simulink model "buckexp9"  (R2024b)
settings: Solver=ode4  StartTime=0.0  StopTime=0.05  FixedStep=1e-8  MaxStep=1e-4  RelTol=1e-3
libraries: spsVoltageMeasurementLib x4, spsSeriesRLCBranchLib x3, spsDiodeLib x1, spsCurrentMeasurementLib x1, spsMosfetLib x1, simulink x1, spsDCVoltageSourceLib x1, sps_lib x1
settings Model: Creator=ece  LastModifiedBy=User
settings SolverCC: AlgebraicLoopSolver=TrustRegion
settings DataIOCC: ReturnWorkspaceOutputs=off
settings DebuggingCC: UnconnectedInputMsg=warning  UnconnectedOutputMsg=warning  UnconnectedLineMsg=warning  ArithmeticOperatorsInVariantConditions=warning
settings ModelReferenceCC: EnableRefExpFcnMdlSchedulingChecks=on
settings SFSimCC: SimUseLocalCustomCode=off  CustomCodeUndefinedFunction=UseInterfaceOnly
settings RTWCC: RTWUseLocalCustomCode=off  GPUComputeCapability=3.5
settings CodeAppCC: StateflowObjectComments=on
settings SimscapeCC: SimscapeNormalizeSystem=off

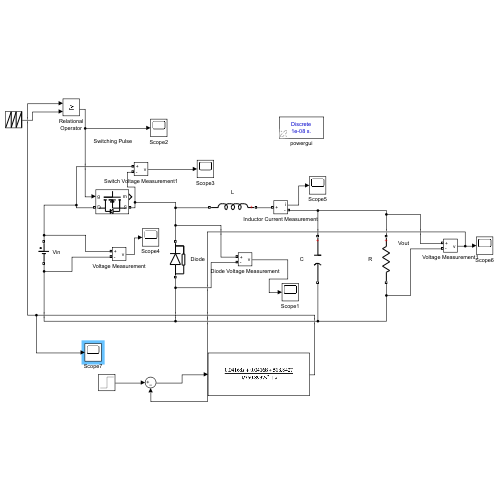
[thumbnail: Simulink's stored preview of the top-level diagram]
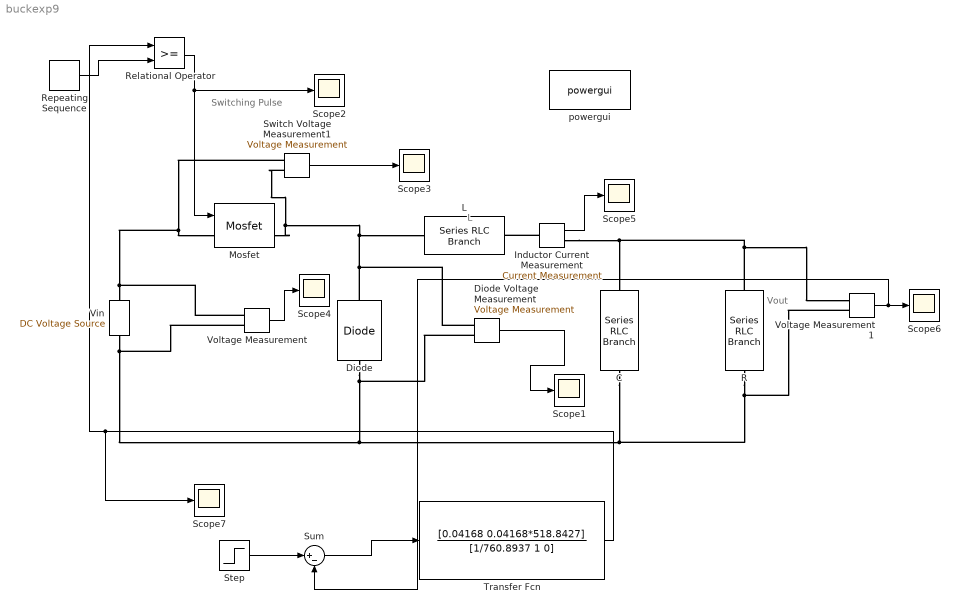
== system buckexp9 ==
  note: Vout
  note: Switching Pulse
  note: L
  "   C" : spsSeriesRLCBranchLib/Series RLC Branch  LConnTagsString=__new0  RConnTagsString=__new0  BranchType=C  Resistance=1  Inductance=1e-3  SetiL0=off  InitialCurrent=0  Capacitance=100e-6  Setx0=off  InitialVoltage=0  Measurements=None
  Diode : spsDiodeLib/Diode  Ron=0.001  Lon=0  Vf=0.8  IC=0  UseSnubber=0  Rs=5e5  Cs=250e-9  Measurements=off
  Diode Voltage Measurement : spsVoltageMeasurementLib/Voltage Measurement  PhasorSimulation=off  OutputType=Complex  PSBequivalent=0
  Inductor Current Measurement : spsCurrentMeasurementLib/Current Measurement  PhasorSimulation=off  OutputType=Complex  PSBequivalent=0
  L : spsSeriesRLCBranchLib/Series RLC Branch  LConnTagsString=__new0  RConnTagsString=__new0  BranchType=L  Resistance=1  Inductance=50e-6  SetiL0=off  InitialCurrent=0  Capacitance=1e-6  Setx0=off  InitialVoltage=0  Measurements=None
  Mosfet : spsMosfetLib/Mosfet  Ron=0.1  Lon=0  Rd=0.01  Vfd=0  IC=0  Rs=1e5  Cs=inf  Measurements=on
  R : spsSeriesRLCBranchLib/Series RLC Branch  LConnTagsString=__new0  RConnTagsString=__new0  BranchType=R  Resistance=2  Inductance=1e-3  SetiL0=off  InitialCurrent=0  Capacitance=1e-6  Setx0=off  InitialVoltage=0  Measurements=None
  Relational Operator : RelationalOperator  OutDataTypeStr=boolean  RndMeth=Simplest  InputSameDT=off
  Repeating Sequence : simulink/Sources/Repeating Sequence  rep_seq_t=[0 1e-5]  rep_seq_y=[0 1]
  Scope{1..7} (7 alike) : Scope
  Step : Step  Time=0.03  Before=10  After=15  SampleTime=0
  Sum : Sum  Inputs=|+-
  Switch Voltage Measurement1 : spsVoltageMeasurementLib/Voltage Measurement  PhasorSimulation=off  OutputType=Complex  PSBequivalent=0
  Transfer Fcn : TransferFcn  Numerator=[0.04168 0.04168*518.8427]  Denominator=[1/760.8937 1 0]
  Vin : spsDCVoltageSourceLib/DC Voltage Source  Amplitude=24  Measurements=None
  Voltage Measurement : spsVoltageMeasurementLib/Voltage Measurement  PhasorSimulation=off  OutputType=Complex  PSBequivalent=0
  Voltage Measurement1 : spsVoltageMeasurementLib/Voltage Measurement  PhasorSimulation=off  OutputType=Complex  PSBequivalent=0
  powergui : sps_lib/powergui  Priority=1  SimulationMode=Discrete  SampleTime=1e-8  frequency=60  Iterations=50  frequencyindice=0  Pbase=100e6  ErrMax=1e-4  UnitsV=kV  UnitsW=MW  buscounter=0  FunctionMessages=off  echomessages=off  EnableUseOfTLC=off  CurrentSourceSwitches=off  DisableSnubberDevices=off  DisableRonSwitches=off  DisableVfSwitches=off  DisplayEquations=off  AutomaticDiscreteSolvers=off  SolverType=Tustin/Backward Euler (TBE)  Interpol=off  ExternalGateDelay=off  methode=off  Ts=100  x0status=blocks  SPID=on  SwTol=0  HookPort=off  NonlinearTolerance=1e-4  nMaxIteration=100  ContinueOnMaxIteration=off  RestoreLinks=warning  ResistiveCurrentMeasurement=off  Frange=[0:2:500]  Ylog=off  Xlog=on  ShowGrid=off  save=off  variable=ZData  structure=0  ZoomFFT=off  StartTime=0.0  cycles=1  DisplayStyle=1  fundamental=60  FreqAxis=off  MaxFrequency=1000  frequencyindicesteady=1  RmsSteady=1  display=off
  wires:
  Relational Operator/1 -> Mosfet/1, Scope2/1
  Repeating Sequence/1 -> Relational Operator/2
  Diode Voltage Measurement/1 -> Scope1/1
  Switch Voltage Measurement1/1 -> Scope3/1
  Voltage Measurement/1 -> Scope4/1
  Inductor Current Measurement/1 -> Scope5/1
  Voltage Measurement1/1 -> Sum/2, Scope6/1
  Sum/1 -> Transfer Fcn/1
  Transfer Fcn/1 -> Scope7/1, Relational Operator/1
  Step/1 -> Sum/1
  connections:
  Diode Voltage Measurement/LConn1 -- Diode/RConn1 -- Mosfet/RConn1 -- Switch Voltage Measurement1/LConn2 -- L/RConn1
  "   C"/RConn1 -- Diode Voltage Measurement/LConn2 -- Diode/LConn1 -- Voltage Measurement/LConn2 -- Vin/LConn1 -- R/RConn1 -- Voltage Measurement1/LConn2
  Inductor Current Measurement/LConn1 -- L/LConn1
  R/LConn1 -- "   C"/LConn1 -- Inductor Current Measurement/RConn1 -- Voltage Measurement1/LConn1
  Vin/RConn1 -- Mosfet/LConn1 -- Switch Voltage Measurement1/LConn1 -- Voltage Measurement/LConn1
